simulink model "myo_sfun_one_myo_imu_emg"  (R2019a)
settings: Solver=ode1  StartTime=0.0  StopTime=inf  FixedStep=0.005  RelTol=1e-3  EnableMultiTasking=on
libraries: neural x1018, myo_lib x2, sldrtlib x1, dspnetwork x1
(part 2 of 12)

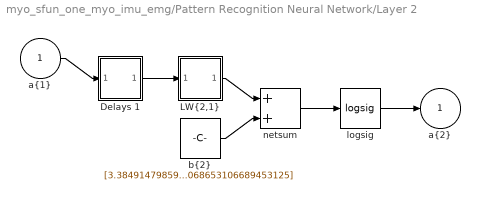
== system myo_sfun_one_myo_imu_emg/Pattern Recognition Neural Network/Layer 2 ==
  "a{1} " : Inport  PortDimensions=8
      mask Display: e = 0.06;c1 = [120 230 180]/255;c2 = ([120 230 180]+0)/(256+128);c3 = ([120 230 180]+128)/(256+128);patch([0 1 1 0],[0 0 1 1],c1);patch([0 1 1 1-e 1-e 0+e],[0 0 1 1-e 0+e 0+e],c2);patch([0 0 1 1-e 0+e 0+e],[0 1 1 1-e 1-e 0+e],c3);plot([0 1 1 0 0],[0 0 1 1 0]);
  Delays 1 : Subsystem
      mask Display: e = 0.06;c1 = [120 150 230]/255;c2 = ([120 150 230]+0)/383;c3 = ([120 150 230]+128)/383;patch([0 1 1 0],[0 0 1 1],c1);patch([0 1 1 1-e 1-e 0+e],[0 0 1 1-e 0+e 0+e],c2);patch([0 0 1 1-e 0+e 0+e],[0 1 1 1-e 1-e 0+e],c3);plot([0 1 1 0 0],[0 0 1 1 0]);disp('0');
  "LW{2,1}" : Subsystem
      mask Display: e = 0.06;c1 = [120 150 230]/255;c2 = ([120 150 230]+0)/383;c3 = ([120 150 230]+128)/383;patch([0 1 1 0],[0 0 1 1],c1);patch([0 1 1 1-e 1-e 0+e],[0 0 1 1-e 0+e 0+e],c2);patch([0 0 1 1-e 0+e 0+e],[0 1 1 1-e 1-e 0+e],c3);plot([0 1 1 0 0],[0 0 1 1 0]);disp('W');
  "b{2}" : Constant  Value=[3.384914798595910045975188040756620466709136962890625;-3.31442931369641513583701453171670436859130859375;3.308455315286777054240019424469210207462310791015625;3.31187322466579647795015262090601027011871337890625;3.280123763624333665944732274510897696018218994140625;-3.291101682623730706467313211760483682155609130859375;-3.3088142324790386084032434155233204364776611328125;-3.26668053382760437131082653650082647800445556640625;-3.267069524518209977514970887568779289722442626953125;-3.2548700464885715888385675498284399509429931640625;-3.2432983611089838404950569383800029754638671875;-3.247445114499055041079600414377637207508087158203125;-3.2276952845823867477292878902517259120941162109375;3.23390971185451281399991785292513668537139892578125;3.21282221349440266777719443780370056629180908203125;-3.2234273144359644192036284948699176311492919921875;3.212914737676046517123040757724083960056304931640625;3.20672161798613242211786200641654431819915771484375;-3.21213044546136483603504530037753283977508544921875;3.17126815566778130772718213847838342189788818359375;3.188203133093212127135984701453708112239837646484375;3.268551936159661774894402697100304067134857177734375;-3.201461175556712834833206215989775955677032470703125;3.1848489393844783279519106145016849040985107421875;3.160476970443632627194574524764902889728546142578125;-3.133411857651147602865648877923376858234405517578125;-3.1384419990674725653434506966732442378997802734375;3.141351487825970512091089403838850557804107666015625;3.088611410227817710705267018056474626064300537109375;3.124771203530135377235410487628541886806488037109375;3.158593462261794826417826698161661624908447265625;-3.097685281819360536559315733029507100582122802734375;-3.103395024396309764824763988144695758819580078125;-3.068142927787715024123826879076659679412841796875;-3.09455517343943942165651606046594679355621337890625;-3.166521227324334830655061523430049419403076171875;3.081835358094869636857993100420571863651275634765625;-3.06495347704127762966663794941268861293792724609375;3.068251509577529123617978257243521511554718017578125;-3.0447183455221011882940729265101253986358642578125;3.0744297160682787506402746657840907573699951171875;3.034020373959843919209333762410096824169158935546875;-2.9569433594943514975739162764512002468109130859375;-3.058287967422655295735012259683571755886077880859375;3.040543609453510764950578959542326629161834716796875;3.011456975851802386756617124774493277072906494140625;-2.9977062241897129979406599886715412139892578125;-3.017719462716960787673770028050057590007781982421875;2.9913301072193423379985688370652496814727783203125;2.982892638598374279723657309659756720066070556640625;2.940139538293412346803279433515854179859161376953125;-2.9776178672232997968194467830471694469451904296875;-2.971894278184042281765186999109573662281036376953125;2.95274818880133960163902884232811629772186279296875;-2.967088646043892108394857132225297391414642333984375;-2.9622633610281781102457898668944835662841796875;2.94661389316522726034008883289061486721038818359375;-2.905020017243308938503787430818192660808563232421875;-2.92516376781045561727978565613739192485809326171875;2.920414910832086707870303143863566219806671142578125;2.92255605313663568978199691628105938434600830078125;2.9339234401006404340250810491852462291717529296875;2.921699788849887458042076104902662336826324462890625;-2.91353630340671632126259282813407480716705322265625;2.851500943653835662416895502246916294097900390625;2.908968021455692554155803009052760899066925048828125;2.93246901734512288584255657042376697063446044921875;2.87569337842594396903450615354813635349273681640625;2.83899853849742189737526132375933229923248291015625;-2.83710006411778437040993594564497470855712890625;2.895166358260958805459495124523527920246124267578125;2.856248595905558573804228217341005802154541015625;-2.83841432730186671307137658004648983478546142578125;2.793091797397988518270040003699250519275665283203125 ...(+50706 chars)]
      mask Display: e = 0.06;c1 = [120 150 230]/255;c2 = ([120 150 230]+0)/383;c3 = ([120 150 230]+128)/383;patch([0 1 1 0],[0 0 1 1],c1);patch([0 1 1 1-e 1-e 0+e],[0 0 1 1-e 0+e 0+e],c2);patch([0 0 1 1-e 0+e 0+e],[0 1 1 1-e 1-e 0+e],c3);plot([0 1 1 0 0],[0 0 1 1 0]);disp('b');
  logsig : neural/Transfer Functions/logsig
      settings: SourceProductName=MATLAB Runtime - Deep Learning Toolbox  SourceProductBaseCode=Missing
  netsum : Sum  Inputs=2  SaturateOnIntegerOverflow=on  InputSameDT=on  OutDataTypeStr=Inherit: Same as first input
      mask Display: e = 0.06;c1 = [120 150 230]/255;c2 = ([120 150 230]+0)/383;c3 = ([120 150 230]+128)/383;patch([0 1 1 0],[0 0 1 1],c1);patch([0 1 1 1-e 1-e 0+e],[0 0 1 1-e 0+e 0+e],c2);patch([0 0 1 1-e 0+e 0+e],[0 1 1 1-e 1-e 0+e],c3);plot([0 1 1 0 0],[0 0 1 1 0]);disp('+');
  "a{2}" : Outport  InitialOutput=[0;0;0;0;0;0;0;0;0;0;0;0;0;0;0;0;0;0;0;0;0;0;0;0;0;0;0;0;0;0;0;0;0;0;0;0;0;0;0;0;0;0;0;0;0;0;0;0;0;0;0;0;0;0;0;0;0;0;0;0;0;0;0;0;0;0;0;0;0;0;0;0;0;0;0;0;0;0;0;0;0;0;0;0;0;0;0;0;0;0;0;0;0;0;0;0;0;0;0;0;0;0;0;0;0;0;0;0;0;0;0;0;0;0;0;0;0;0;0;0;0;0;0;0;0;0;0;0;0;0;0;0;0;0;0;0;0;0;0;0;0;0;0;0;0;0;0;0;0;0;0;0;0;0;0;0;0;0;0;0;0;0;0;0;0;0;0;0;0;0;0;0;0;0;0;0;0;0;0;0;0;0;0;0;0;0;0;0;0;0;0;0;0;0;0;0;0;0;0;0;0;0;0;0;0;0;0;0;0;0;0;0;0;0;0;0;0;0;0;0;0;0;0;0;0;0;0;0;0;0;0;0;0;0;0;0;0;0;0;0;0;0;0;0;0;0;0;0;0;0;0;0;0;0;0;0;0;0;0;0;0;0;0;0;0;0;0;0;0;0;0;0;0;0;0;0;0;0;0;0;0;0;0;0;0;0;0;0;0;0;0;0;0;0;0;0;0;0;0;0;0;0;0;0;0;0;0;0;0;0;0;0;0;0;0;0;0;0;0;0;0;0;0;0;0;0;0;0;0;0;0;0;0;0;0;0;0;0;0;0;0;0;0;0;0;0;0;0;0;0;0;0;0;0;0;0;0;0;0;0;0;0;0;0;0;0;0;0;0;0;0;0;0;0;0;0;0;0;0;0;0;0;0;0;0;0;0;0;0;0;0;0;0;0;0;0;0;0;0;0;0;0;0;0;0;0;0;0;0;0;0;0;0;0;0;0;0;0;0;0;0;0;0;0;0;0;0;0;0;0;0;0;0;0;0;0;0;0;0;0;0;0;0;0;0;0;0;0;0;0;0;0;0;0;0;0;0;0;0;0;0;0;0;0;0;0;0;0;0;0;0;0;0;0;0;0;0;0;0;0;0;0;0;0;0;0;0;0;0;0;0;0;0;0;0;0;0;0;0;0;0;0;0;0;0;0;0;0;0;0;0;0;0;0;0;0;0;0;0;0;0;0;0;0;0;0;0;0;0;0;0;0;0;0;0;0;0;0;0;0;0;0;0;0;0;0;0;0;0;0;0;0;0;0;0;0;0;0;0;0;0;0;0;0;0;0;0;0;0;0;0;0;0;0;0;0;0;0;0;0;0;0;0;0;0;0;0;0;0;0;0;0;0;0;0;0;0;0;0;0;0;0;0;0;0;0;0;0;0;0;0;0;0;0;0;0;0;0;0;0;0;0;0;0;0;0;0;0;0;0;0;0;0;0;0;0;0;0;0;0;0;0;0;0;0;0;0;0;0;0;0;0;0;0;0;0;0;0;0;0;0;0;0;0;0;0;0;0;0;0;0;0;0;0;0;0;0;0;0;0;0;0;0;0;0;0;0;0;0;0;0;0;0;0;0;0;0;0;0;0;0;0;0;0;0;0;0;0;0;0;0;0;0;0;0;0;0;0;0;0;0;0;0;0;0;0;0;0;0;0;0;0;0;0;0;0;0;0;0;0;0;0;0;0;0;0;0;0;0;0;0;0;0;0;0;0;0;0;0;0;0;0;0;0;0;0;0;0;0;0;0;0;0;0;0;0;0;0;0;0;0;0;0;0;0;0;0;0;0;0;0;0;0;0;0;0;0;0;0;0;0;0;0;0;0;0;0;0;0;0;0;0;0;0;0;0;0;0;0;0;0;0;0;0;0;0;0;0;0;0;0;0;0;0;0;0;0;0;0;0;0;0;0;0;0;0;0;0;0;0;0;0;0;0;0;0;0;0;0;0;0;0;0;0;0;0;0;0;0;0;0;0;0;0;0;0;0;0;0;0;0;0;0;0;0;0;0;0;0;0;0;0;0;0;0;0;0;0;0;0;0;0;0;0;0;0;0;0;0;0;0;0;0;0;0;0;0;0;0;0;0;0;0;0;0;0;0;0;0;0;0;0;0;0;0;0;0;0;0;0;0;0;0;0;0;0;0;0;0;0;0;0;0;0;0;0;0;0;0;0;0;0;0;0;0;0;0;0;0;0;0;0;0;0;0;0;0;0;0;0;0;0;0;0;0;0;0;0;0;0;0;0;0;0;0;0;0;0;0;0]
      mask Display: e = 0.06;c1 = [120 230 180]/255;c2 = ([120 230 180]+0)/(256+128);c3 = ([120 230 180]+128)/(256+128);patch([0 1 1 0],[0 0 1 1],c1);patch([0 1 1 1-e 1-e 0+e],[0 0 1 1-e 0+e 0+e],c2);patch([0 0 1 1-e 0+e 0+e],[0 1 1 1-e 1-e 0+e],c3);plot([0 1 1 0 0],[0 0 1 1 0]);
  wires:
  logsig/1 -> "a{2}"/1
  netsum/1 -> logsig/1
  "b{2}"/1 -> netsum/2
  "LW{2,1}"/1("lz{2,1}") -> netsum/1
  Delays 1/1("pd{2,1}") -> "LW{2,1}"/1("ad{2,1}")
  "a{1} "/1 -> Delays 1/1("p{2}")
